simulink model "dq0_double"  (R2020b)
settings: Solver=FixedStepAuto  StartTime=0.0  StopTime=tStop  FixedStep=tStep  RelTol=1e-3
values from neighbouring files (symbols this model uses):
  amp = [0, amplitude]    [dq_double_main.m]
  f_c = 50    [dq_double_main.m]
  freq = [f_meas f_meas]    [dq_double_main.m]
  L_a = 27e-3    (= 0.027)    [dq_double_main.m]
  L_g = 50e-3    (= 0.05)    [dq_double_main.m]
  phase = [1/2*pi 1/2*pi]    [dq_double_main.m]
  R_a = 15    [dq_double_main.m]
  R_g = 20    [dq_double_main.m]
libraries: powerlib x29, SimplusGT x6
settings Model: Creator=kacper  LastModifiedBy=kacper

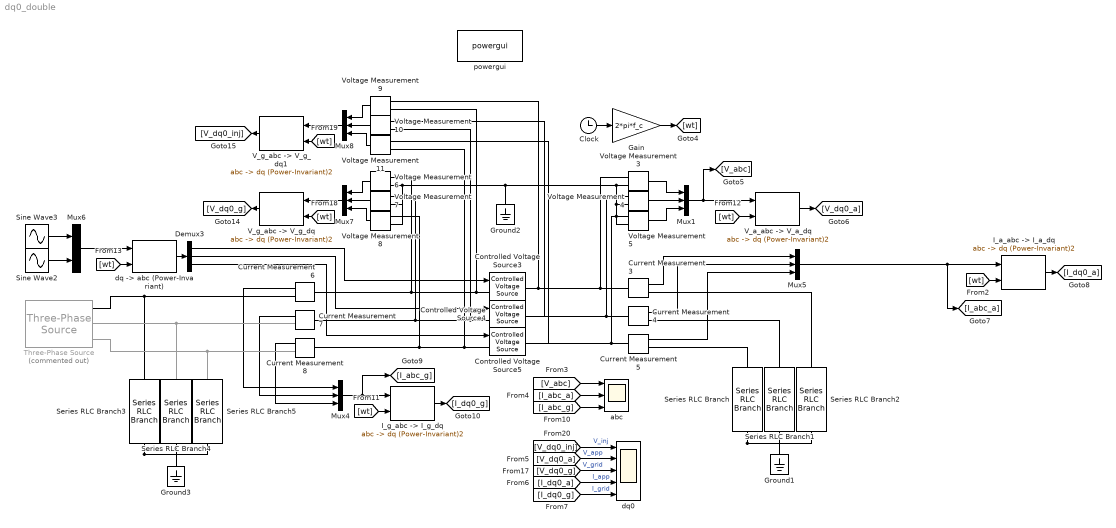
== system dq0_double ==
  Clock : Clock
  Controlled Voltage Source3 : powerlib/Electrical Sources/Controlled Voltage Source  Initialize=on  Source_Type=AC  Amplitude=0  Phase=0  Frequency=0  Measurements=None
  Controlled Voltage Source4 : powerlib/Electrical Sources/Controlled Voltage Source  Initialize=on  Source_Type=AC  Amplitude=0  Phase=0  Frequency=0  Measurements=None
  Controlled Voltage Source5 : powerlib/Electrical Sources/Controlled Voltage Source  Initialize=on  Source_Type=AC  Amplitude=0  Phase=0  Frequency=0  Measurements=None
  Current Measurement{3..8} (6 alike) : powerlib/Measurements/Current Measurement  PhasorSimulation=off  OutputType=Complex  PSBequivalent=0
  Demux3 : Demux  Outputs=3
  Gain : Gain  Gain=2*pi*f_c
  Ground1 : powerlib/Elements/Ground  LConnTagsString=a
  Ground2 : powerlib/Elements/Ground  LConnTagsString=a
  Ground3 : powerlib/Elements/Ground  LConnTagsString=a
  "I_a_abc -> I_a_dq" : SimplusGT/Grid-Following Voltage-Source Inverter (dq-Frame System Object)/abc -> dq (Power-Invariant)2  SystemSampleTime=-1  VariantActivationTime=update diagram  Latency=0  AutoFrameSizeCalculation=off
  "I_g_abc -> I_g_dq" : SimplusGT/Grid-Following Voltage-Source Inverter (dq-Frame System Object)/abc -> dq (Power-Invariant)2  SystemSampleTime=-1  VariantActivationTime=update diagram  Latency=0  AutoFrameSizeCalculation=off
  Mux{1,4..5,7..8} (5 alike) : Mux  Inputs=3
  Mux6 : Mux  Inputs=2
  Series RLC Branch : powerlib/Elements/Series RLC Branch  LConnTagsString=__new0  RConnTagsString=__new0  BranchType=RL  Resistance=R_a  Inductance=L_a  SetiL0=off  InitialCurrent=0  Capacitance=1e-6  Setx0=off  InitialVoltage=0  Measurements=None
  Series RLC Branch1 : powerlib/Elements/Series RLC Branch  LConnTagsString=__new0  RConnTagsString=__new0  BranchType=RL  Resistance=R_a  Inductance=L_a  SetiL0=off  InitialCurrent=0  Capacitance=1e-6  Setx0=off  InitialVoltage=0  Measurements=None
  Series RLC Branch2 : powerlib/Elements/Series RLC Branch  LConnTagsString=__new0  RConnTagsString=__new0  BranchType=RL  Resistance=R_a  Inductance=L_a  SetiL0=off  InitialCurrent=0  Capacitance=1e-6  Setx0=off  InitialVoltage=0  Measurements=None
  Series RLC Branch3 : powerlib/Elements/Series RLC Branch  LConnTagsString=__new0  RConnTagsString=__new0  BranchType=RL  Resistance=R_g  Inductance=L_g  SetiL0=off  InitialCurrent=0  Capacitance=1e-6  Setx0=off  InitialVoltage=0  Measurements=None
  Series RLC Branch4 : powerlib/Elements/Series RLC Branch  LConnTagsString=__new0  RConnTagsString=__new0  BranchType=RL  Resistance=R_g  Inductance=L_g  SetiL0=off  InitialCurrent=0  Capacitance=1e-6  Setx0=off  InitialVoltage=0  Measurements=None
  Series RLC Branch5 : powerlib/Elements/Series RLC Branch  LConnTagsString=__new0  RConnTagsString=__new0  BranchType=RL  Resistance=R_g  Inductance=L_g  SetiL0=off  InitialCurrent=0  Capacitance=1e-6  Setx0=off  InitialVoltage=0  Measurements=None
  Sine Wave2 : Sin  Amplitude=amp(1,2)  Frequency=2*pi*freq(1,2)  Phase=phase(1,2)  SampleTime=0
  Sine Wave3 : Sin  Amplitude=amp(1,1)  Frequency=2*pi*freq(1,1)  Phase=phase(1,1)  SampleTime=0
  Three-Phase Source : powerlib/Electrical Sources/Three-Phase Source  Commented=on  InternalConnection=Yg  VoltagePhases=off  Voltage=400e3  PhaseAngle=0  Voltage_phases=[25e3 25e3 25e3]/sqrt(3)  PhaseAngles_phases=[0 -120 +120]  Frequency=f_c  NonIdealSource=off  SpecifyImpedance=off  Resistance=0.8929  Inductance=16.58e-3  ShortCircuitLevel=100e6  BaseVoltage=25e3  XRratio=7  BusType=swing  Pref=10e3  Qref=0  Prefabc=[10e3, 10e3, 10e3]  Qrefabc=[0, 0, 0]  Qmin=-inf  Qmax=inf
  "V_a_abc -> V_a_dq" : SimplusGT/Grid-Following Voltage-Source Inverter (dq-Frame System Object)/abc -> dq (Power-Invariant)2  SystemSampleTime=-1  VariantActivationTime=update diagram  Latency=0  AutoFrameSizeCalculation=off
  "V_g_abc -> V_g_dq" : SimplusGT/Grid-Following Voltage-Source Inverter (dq-Frame System Object)/abc -> dq (Power-Invariant)2  SystemSampleTime=-1  VariantActivationTime=update diagram  Latency=0  AutoFrameSizeCalculation=off
  "V_g_abc -> V_g_dq1" : SimplusGT/Grid-Following Voltage-Source Inverter (dq-Frame System Object)/abc -> dq (Power-Invariant)2  SystemSampleTime=-1  VariantActivationTime=update diagram  Latency=0  AutoFrameSizeCalculation=off
  Voltage Measurement{3..11} (9 alike) : powerlib/Measurements/Voltage Measurement  PhasorSimulation=off  OutputType=Complex  PSBequivalent=0
  abc : Scope  NumInputPorts=3
  "dq -> abc (Power-Invariant)" : SimplusGT/dq -> abc (Power-Invariant)  SystemSampleTime=-1  VariantActivationTime=update diagram  Latency=0  AutoFrameSizeCalculation=off
  dq0 : Scope  NumInputPorts=5
  powergui : powerlib/powergui  Priority=1  SimulationMode=Continuous  SampleTime=50e-6  frequency=60  Iterations=50  frequencyindice=0  Pbase=100e6  ErrMax=1e-4  UnitsV=kV  UnitsW=MW  buscounter=0  FunctionMessages=off  echomessages=off  EnableUseOfTLC=off  CurrentSourceSwitches=off  DisableSnubberDevices=off  DisableRonSwitches=off  DisableVfSwitches=off  DisplayEquations=off  AutomaticDiscreteSolvers=off  SolverType=Tustin/Backward Euler (TBE)  Interpol=off  ExternalGateDelay=off  methode=off  Ts=100  x0status=blocks  SPID=on  SwTol=0  HookPort=off  NonlinearTolerance=1e-4  nMaxIteration=100  ContinueOnMaxIteration=off  RestoreLinks=warning  ResistiveCurrentMeasurement=off  Frange=[0:2:500]  Ylog=off  Xlog=on  ShowGrid=off  save=off  variable=ZData  structure=0  ZoomFFT=off  StartTime=0.0  cycles=1  DisplayStyle=1  fundamental=60  FreqAxis=off  MaxFrequency=1000  frequencyindicesteady=1  RmsSteady=1  display=off
  wires:
  Clock/1 -> Gain/1
  Gain/1 -> [wt]
  [wt] -> "I_g_abc -> I_g_dq"/2
  [wt] -> "V_a_abc -> V_a_dq"/2
  Sine Wave3/1 -> Mux6/1
  Current Measurement6/1 -> Mux4/1
  Mux4/1 -> "I_g_abc -> I_g_dq"/1, [I_abc_g]
  [I_dq0_g] -> dq0/5  "I_grid"
  "V_g_abc -> V_g_dq"/1 -> [V_dq0_g]
  [V_dq0_g] -> dq0/3  "V_grid"
  Voltage Measurement9/1 -> Mux8/1
  [I_abc_g] -> abc/3
  Voltage Measurement3/1 -> Mux1/1
  "I_g_abc -> I_g_dq"/1 -> [I_dq0_g]
  Voltage Measurement6/1 -> Mux7/1
  "dq -> abc (Power-Invariant)"/1 -> Demux3/1
  [wt] -> "dq -> abc (Power-Invariant)"/2
  "V_a_abc -> V_a_dq"/1 -> [V_dq0_a]
  "I_a_abc -> I_a_dq"/1 -> [I_dq0_a]
  [wt] -> "I_a_abc -> I_a_dq"/2
  [I_dq0_a] -> dq0/4  "I_app"
  Voltage Measurement4/1 -> Mux1/2
  Voltage Measurement8/1 -> Mux7/3
  Mux7/1 -> "V_g_abc -> V_g_dq"/1
  Mux5/1 -> "I_a_abc -> I_a_dq"/1, [I_abc_a]
  [wt] -> "V_g_abc -> V_g_dq"/2
  Voltage Measurement11/1 -> Mux8/3
  Current Measurement3/1 -> Mux5/1
  Mux8/1 -> "V_g_abc -> V_g_dq1"/1
  Voltage Measurement10/1 -> Mux8/2
  Current Measurement8/1 -> Mux4/3
  Sine Wave2/1 -> Mux6/2
  "V_g_abc -> V_g_dq1"/1 -> [V_dq0_inj]
  Demux3/1 -> Controlled Voltage Source3/1
  [V_dq0_a] -> dq0/2  "V_app"
  [V_dq0_inj] -> dq0/1  "V_inj"
  Mux6/1 -> "dq -> abc (Power-Invariant)"/1
  Demux3/2 -> Controlled Voltage Source4/1
  Voltage Measurement7/1 -> Mux7/2
  [wt] -> "V_g_abc -> V_g_dq1"/2
  Mux1/1 -> "V_a_abc -> V_a_dq"/1, [V_abc]
  Current Measurement7/1 -> Mux4/2
  [I_abc_a] -> abc/2
  Current Measurement4/1 -> Mux5/2
  [V_abc] -> abc/1
  Voltage Measurement5/1 -> Mux1/3
  Demux3/3 -> Controlled Voltage Source5/1
  Current Measurement5/1 -> Mux5/3
  connections:
  Voltage Measurement8/LConn1 -- Current Measurement8/LConn1 -- Voltage Measurement11/LConn2 -- Controlled Voltage Source5/LConn1
  Controlled Voltage Source4/LConn1 -- Voltage Measurement10/LConn2 -- Voltage Measurement7/LConn1 -- Current Measurement7/LConn1
  Voltage Measurement6/LConn2 -- Ground2/LConn1 -- Voltage Measurement5/LConn2 -- Voltage Measurement4/LConn2 -- Voltage Measurement3/LConn2 -- Voltage Measurement8/LConn2 -- Voltage Measurement7/LConn2
  Controlled Voltage Source3/RConn1 -- Voltage Measurement9/LConn1 -- Current Measurement3/LConn1 -- Voltage Measurement3/LConn1
  Voltage Measurement6/LConn1 -- Current Measurement6/LConn1 -- Voltage Measurement9/LConn2 -- Controlled Voltage Source3/LConn1
  Voltage Measurement4/LConn1 -- Voltage Measurement10/LConn1 -- Controlled Voltage Source4/RConn1 -- Current Measurement4/LConn1
  Voltage Measurement5/LConn1 -- Voltage Measurement11/LConn1 -- Controlled Voltage Source5/RConn1 -- Current Measurement5/LConn1
  Current Measurement6/RConn1 -- Series RLC Branch3/LConn1 -- Three-Phase Source/RConn1
  Series RLC Branch/RConn1 -- Ground1/LConn1 -- Series RLC Branch1/RConn1 -- Series RLC Branch2/RConn1
  Current Measurement3/RConn1 -- Series RLC Branch2/LConn1
  Current Measurement4/RConn1 -- Series RLC Branch1/LConn1
  Current Measurement5/RConn1 -- Series RLC Branch/LConn1
  Three-Phase Source/RConn2 -- Series RLC Branch4/LConn1 -- Current Measurement7/RConn1
  Three-Phase Source/RConn3 -- Series RLC Branch5/LConn1 -- Current Measurement8/RConn1
  Series RLC Branch3/RConn1 -- Ground3/LConn1 -- Series RLC Branch4/RConn1 -- Series RLC Branch5/RConn1
